simulink model "test_sim"  (R2023b)
settings: Solver=FixedStepAuto  StartTime=0.0  StopTime=10000  FixedStep=step_T  RelTol=1e-3
InitFcn:
  | run('pam_test')
values from neighbouring files (symbols this model uses):
  step_T = 0.01    [pam_test.m]
  tau = 1/max(eig(pam.S))    [S2_calculate_parameters.m]    (also in pam_test.m = 0.5)
  w_0 = 0.37    [pam_test.m]
  x_0 = 0.016    [pam_test.m]
  y_0 = 0.11    [pam_test.m]
  z_0 = 0.3    [pam_test.m]
settings Model: Creator=admin  LastModifiedBy=admin

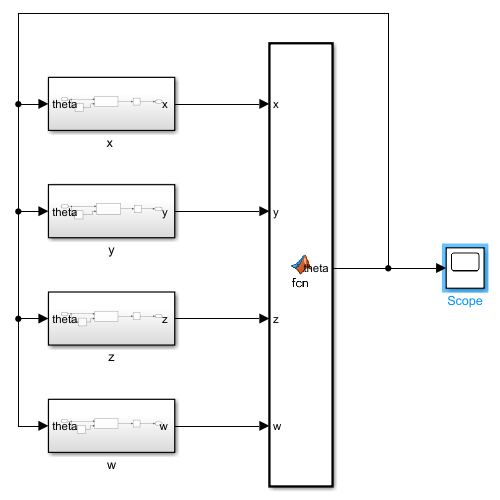
[thumbnail: Simulink's stored preview of the top-level diagram]
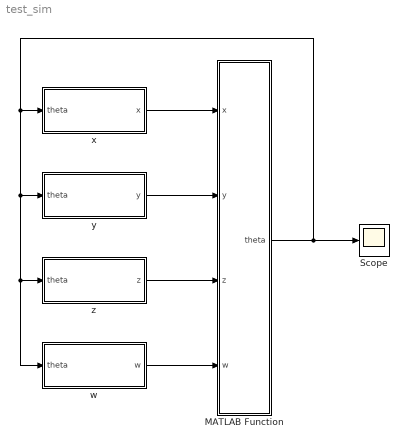
== system test_sim ==
  MATLAB Function : MATLAB Function  TreatAsAtomicUnit=on
  Scope : Scope
  w : Subsystem
  "x " : Subsystem
  y : Subsystem
  z : Subsystem
  wires:
  "x "/1("x ") -> MATLAB Function/1(x)
  y/1("y ") -> MATLAB Function/2(y)
  z/1("z ") -> MATLAB Function/3(z)
  w/1("w ") -> MATLAB Function/4(w)
  MATLAB Function/1(theta) -> Scope/1, w/1(theta), z/1(theta), y/1(theta), "x "/1(theta)

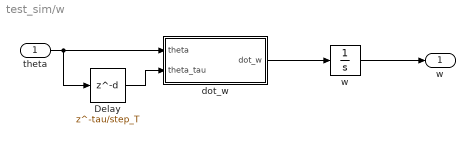
== system test_sim/w ==
  theta : Inport
  Delay : Delay  DelayLength=tau/step_T  InitialCondition=0
  dot_w : MATLAB Function  TreatAsAtomicUnit=on
  w : Integrator  InitialCondition=w_0
  "w " : Outport
  wires:
  dot_w/1(dot_w) -> w/1
  w/1 -> "w "/1
  theta/1 -> Delay/1, dot_w/1(theta)
  Delay/1 -> dot_w/2(theta_tau)

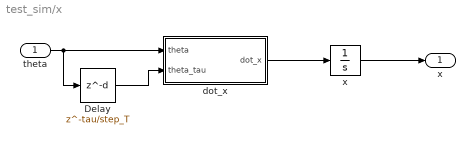
== system test_sim/x  ==
  theta : Inport
  Delay : Delay  DelayLength=tau/step_T  InitialCondition=0
  dot_x : MATLAB Function  TreatAsAtomicUnit=on
  x : Integrator  InitialCondition=x_0
  "x " : Outport
  wires:
  dot_x/1(dot_x) -> x/1
  x/1 -> "x "/1
  theta/1 -> Delay/1, dot_x/1(theta)
  Delay/1 -> dot_x/2(theta_tau)

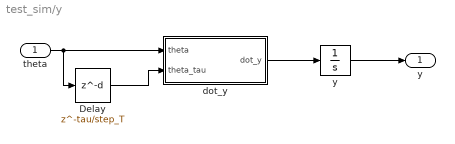
== system test_sim/y ==
  theta : Inport
  Delay : Delay  DelayLength=tau/step_T  InitialCondition=0
  dot_y : MATLAB Function  TreatAsAtomicUnit=on
  y : Integrator  InitialCondition=y_0
  "y " : Outport
  wires:
  dot_y/1(dot_y) -> y/1
  y/1 -> "y "/1
  theta/1 -> Delay/1, dot_y/1(theta)
  Delay/1 -> dot_y/2(theta_tau)

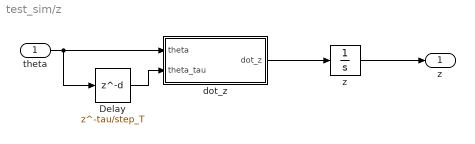
== system test_sim/z ==
  theta : Inport
  Delay : Delay  DelayLength=tau/step_T  InitialCondition=0
  dot_z : MATLAB Function  TreatAsAtomicUnit=on
  z : Integrator  InitialCondition=z_0
  "z " : Outport
  wires:
  dot_z/1(dot_z) -> z/1
  z/1 -> "z "/1
  theta/1 -> Delay/1, dot_z/1(theta)
  Delay/1 -> dot_z/2(theta_tau)

== matlab function test_sim/y/dot_y ==
  data: theta input; theta_tau input; dot_y output size=1; pam parameter
function dot_y = fcn(theta,theta_tau,pam)

x = theta(1);
y = theta(2);
z = theta(3);
w = theta(4);

x_tau = theta_tau(1);
y_tau = theta_tau(2);
z_tau = theta_tau(3);
w_tau = theta_tau(4);

dot_y =- pam.b_1*y-pam.b_2+pam.b_3*x*(pam.N-(x_tau-z_tau));

== matlab function test_sim/x /dot_x ==
  data: theta input; theta_tau input; dot_x output size=1; pam parameter
function dot_x = fcn(theta,theta_tau,pam)

x = theta(1);
y = theta(2);
z = theta(3);
w = theta(4);

x_tau = theta_tau(1);
y_tau = theta_tau(2);
z_tau = theta_tau(3);
w_tau = theta_tau(4);

dot_x = pam.a_1*x*(1-x_tau/pam.M)-pam.a_2*(y_tau+z_tau)-pam.d_3*w_tau;

== matlab function test_sim/z/dot_z ==
  data: theta input; theta_tau input; dot_z output size=1; pam parameter
function dot_z = fcn(theta,theta_tau,pam)

x = theta(1);
y = theta(2);
z = theta(3);
w = theta(4);

x_tau = theta_tau(1);
y_tau = theta_tau(2);
z_tau = theta_tau(3);
w_tau = theta_tau(4);

dot_z =pam.c_1*z*(pam.c_2*x_tau-pam.c_3);

== matlab function test_sim/w/dot_w ==
  data: theta input; theta_tau input; dot_w output size=1; pam parameter
function dot_w = fcn(theta,theta_tau,pam)

x = theta(1);
y = theta(2);
z = theta(3);
w = theta(4);

x_tau = theta_tau(1);
y_tau = theta_tau(2);
z_tau = theta_tau(3);
w_tau = theta_tau(4);

dot_w = pam.d_1*x-pam.d_2*w+pam.K*(w-w_tau);

== matlab function test_sim/MATLAB Function ==
  data: x input; theta output size=[4,1]; y input; z input; w input
function theta = fcn(x,y,z,w)

theta = [x;y;z;w];
